simulink model "FG_costante"  (R2020a)
settings: Solver=VariableStepAuto  StartTime=0.0  StopTime=10.0  RelTol=1e-3
values from neighbouring files (symbols this model uses):
  g = 9.81    [dati_tesi_modellosimulink.m]
  L = 0.3    [dati_tesi_modellosimulink.m]
  Lc = L/2    (= 0.15)    [dati_tesi_modellosimulink.m]
  M = 4    [dati_tesi_modellosimulink.m]
  mc = 0    [dati_tesi_modellosimulink.m]
libraries: fuzblock x7, simulink x5, simulink_extras x2
settings Model: Creator=laura  LastModifiedBy=laura

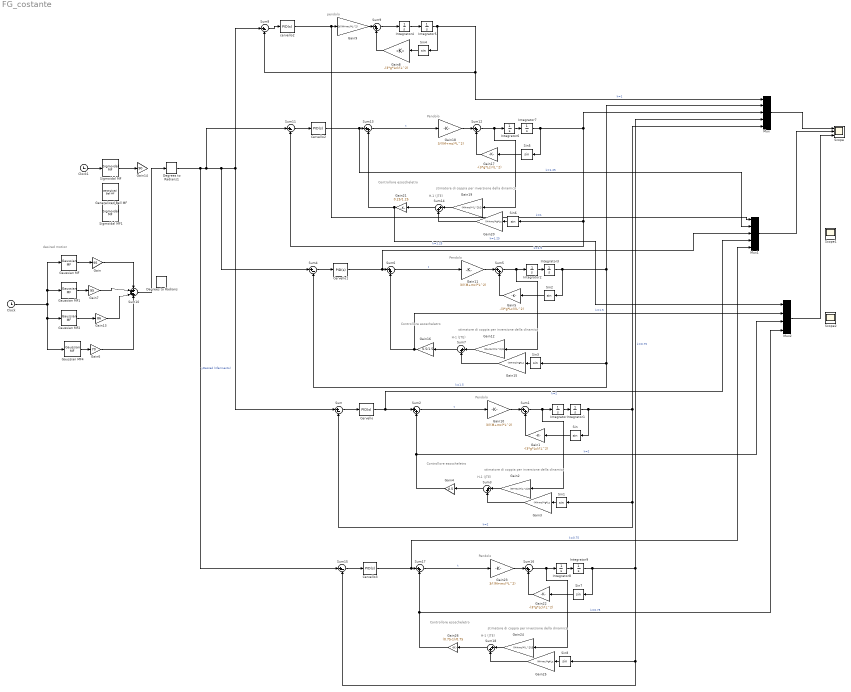
== system FG_costante ==
  note: Controllore esoscheletro
  note: stimatore di coppia per inversione della dinamica
  note: pendolo
  note: Pendolo
  note: H-1 (JTE)
  note: desired motion
  note: Pendolo
  note: H-1 (JTE)
  note: Controllore esoscheletro
  note: stimatore di coppia per inversione della dinamica
  note: Pendolo
  note: H-1 (JTE)
  note: Controllore esoscheletro
  note: stimatore di coppia per inversione della dinamica
  note: Pendolo
  note: H-1 (JTE)
  note: Controllore esoscheletro
  note: stimatore di coppia per inversione della dinamica
  Cervello{,1..3} (4 alike) : simulink/Continuous/PID Controller  Controller=PID  Form=Parallel  TimeDomain=Continuous-time  UseExternalTs=off  SampleTime=-1  IntegratorMethod=Forward Euler  FilterMethod=Forward Euler  ControllerParametersSource=internal  P=20.396  I=105.7651  D=6.3413  UseFilter=on  N=150.7964  TunerSelectOption=Transfer Function Based (PID Tuner App)  InitialConditionSource=internal  InitialConditionForIntegrator=0  InitialConditionForFilter=0  DifferentiatorICPrevScaledInput=0  ExternalReset=none  TrackingMode=off  Kt=1  LimitOutput=off  UpperSaturationLimit=inf  LowerSaturationLimit=-inf  LinearizeAsGain=on  AntiWindupMode=none  Kb=1  POutMin=[]  POutMax=[]  IOutMin=[]  IOutMax=[]  DOutMin=[]  DOutMax=[]  NOutMin=[]  NOutMax=[]  SumOutMin=[]  SumOutMax=[]  SaturationOutMin=[]  SaturationOutMax=[]  PParamMin=[]  PParamMax=[]  IParamMin=[]  IParamMax=[]  DParamMin=[]  DParamMax=[]  NParamMin=[]  NParamMax=[]  KbParamMin=[]  KbParamMax=[]  KtParamMin=[]  KtParamMax=[]  KbOutMin=[]  KbOutMax=[]  KtOutMin=[]  KtOutMax=[]  IntegratorOutMin=[]  IntegratorOutMax=[]  FilterOutMin=[]  FilterOutMax=[]  SumI1OutMin=[]  SumI1OutMax=[]  SumI2OutMin=[]  SumI2OutMax=[]  SumI3OutMin=[]  SumI3OutMax=[]  SumI4OutMin=[]  SumI4OutMax=[]  SumDOutMin=[]  SumDOutMax=[]  DifferentiatorOutMin=[]  DifferentiatorOutMax=[]  FilterDiffOutCoefMin=[]  FilterDiffOutCoefMax=[]  ReciprocalOutMin=[]  ReciprocalOutMax=[]  SumDenOutMin=[]  SumDenOutMax=[]  SumNumOutMin=[]  SumNumOutMax=[]  DivideOutMin=[]  DivideOutMax=[]  UdiffTsProdOutMin=[]  UdiffTsProdOutMax=[]  NTsProdOutMin=[]  NTsProdOutMax=[]  UintegralTsProdOutMin=[]  UintegralTsProdOutMax=[]  UngainTsProdOutMin=[]  UngainTsProdOutMax=[]  IntegratorContinuousStateAttributes=''  IntegratorStateMustResolveToSignalObject=off  IntegratorRTWStateStorageClass=Auto  FilterContinuousStateAttributes=''  FilterStateMustResolveToSignalObject=off  FilterRTWStateStorageClass=Auto  ParallelPVariant=InternalParameters  IdealPVariant=Disabled  IVariant=InternalParameters  DVariant=InternalParameters  IntegratorVariant=Continuous  SatVariant=Disabled  AWVariant=Passthrough  PCopyVariant=Disabled  TRVariant=Disabled  FdbkBlocksVariant=Forward  IdealPFdbkVariant=Disabled  SatFdbkVariant=Disabled  DerivativeFilterVariant=ContFilter  NVariant=InternalParameters  NCopyVariant=Disabled  FilterICVariant=InternalICsFilter  IntegratorICVariant=InternalICs  ExternalResetVariant=Disabled  TRSumVariant=Passthrough  SumFdbkVariant=Disabled  SumVariant=Sum_PID  TsampFilterVariant=InternalTs  TsampNgainVariant=Passthrough  TsampIntegralVariant=Passthrough
  Clock : Clock
  Clock1 : Clock
  Degrees to Radians : simulink_extras/Transformations/Degrees to Radians
  Degrees to Radians1 : simulink_extras/Transformations/Degrees to Radians
  Gain : Gain  Gain=95
  Gain{1,5,8,17,22} (5 alike) : Gain  Gain=-(3*g*Lc)/(L^2)
  Gain{9..11,18,23} (5 alike) : Gain  Gain=3/((M+mc)*L^2)
  Gain{2,12,19,24} (4 alike) : Gain  Gain=(M+mc)*(L^2)/3
  Gain13 : Gain  Gain=86
  Gain14 : Gain  Gain=90
  Gain{3,15,20,25} (4 alike) : Gain  Gain=(M+mc)*g*Lc
  Gain16 : Gain  Gain=0.5/1.5
  Gain21 : Gain  Gain=0.25/1.25
  Gain26 : Gain  Gain=(0.75-1)/0.75
  Gain4 : Gain  Gain=0.5
  Gain6 : Gain  Gain=70
  Gain7 : Gain  Gain=95
  Gaussian MF : fuzblock/Membership  Functions/Gaussian MF  sigma=0.4  mu=1.78
      settings: SourceProductBaseCode=FL
  Gaussian MF1 : fuzblock/Membership  Functions/Gaussian MF  sigma=0.4  mu=7
      settings: SourceProductBaseCode=FL
  Gaussian MF2 : fuzblock/Membership  Functions/Gaussian MF  sigma=0.38  mu=3.42
      settings: SourceProductBaseCode=FL
  Gaussian MF4 : fuzblock/Membership  Functions/Gaussian MF  sigma=0.32  mu=2.63
      settings: SourceProductBaseCode=FL
  Generalized Bell MF : fuzblock/Membership  Functions/Generalized Bell MF  a=1.5  b=4  c=6
      settings: SourceProductBaseCode=FL
  Integrator{,1..9} (10 alike) : Integrator
  Mux : Mux  Inputs=5
  Mux1 : Mux  Inputs=5
  Mux2 : Mux
  Scope : Scope  NumInputPorts=3
  Scope1 : Scope
  Scope2 : Scope
  Sigmoidal MF : fuzblock/Membership  Functions/Sigmoidal MF  a=4  c=5
      settings: SourceProductBaseCode=FL
  Sigmoidal MF1 : fuzblock/Membership  Functions/Sigmoidal MF  a=-4  c=5
      settings: SourceProductBaseCode=FL
  Sin{,1..8} (9 alike) : Trigonometry
  Sum{,4,8,11,15} (5 alike) : Sum  Inputs=|+-
  Sum{1..3,5..7,9,12..14,16..18} (13 alike) : Sum  Inputs=|++
  Sum10 : Sum  Inputs=++++
  cervello2 : simulink/Continuous/PID Controller  Controller=PID  Form=Parallel  TimeDomain=Continuous-time  UseExternalTs=off  SampleTime=-1  IntegratorMethod=Forward Euler  FilterMethod=Forward Euler  ControllerParametersSource=internal  P=20.396  I=105.7651  D=6.3413  UseFilter=on  N=150.7964  TunerSelectOption=Transfer Function Based (PID Tuner App)  InitialConditionSource=internal  InitialConditionForIntegrator=0  InitialConditionForFilter=0  DifferentiatorICPrevScaledInput=0  ExternalReset=none  TrackingMode=off  Kt=1  LimitOutput=off  UpperSaturationLimit=inf  LowerSaturationLimit=-inf  LinearizeAsGain=on  AntiWindupMode=none  Kb=1  POutMin=[]  POutMax=[]  IOutMin=[]  IOutMax=[]  DOutMin=[]  DOutMax=[]  NOutMin=[]  NOutMax=[]  SumOutMin=[]  SumOutMax=[]  SaturationOutMin=[]  SaturationOutMax=[]  PParamMin=[]  PParamMax=[]  IParamMin=[]  IParamMax=[]  DParamMin=[]  DParamMax=[]  NParamMin=[]  NParamMax=[]  KbParamMin=[]  KbParamMax=[]  KtParamMin=[]  KtParamMax=[]  KbOutMin=[]  KbOutMax=[]  KtOutMin=[]  KtOutMax=[]  IntegratorOutMin=[]  IntegratorOutMax=[]  FilterOutMin=[]  FilterOutMax=[]  SumI1OutMin=[]  SumI1OutMax=[]  SumI2OutMin=[]  SumI2OutMax=[]  SumI3OutMin=[]  SumI3OutMax=[]  SumI4OutMin=[]  SumI4OutMax=[]  SumDOutMin=[]  SumDOutMax=[]  DifferentiatorOutMin=[]  DifferentiatorOutMax=[]  FilterDiffOutCoefMin=[]  FilterDiffOutCoefMax=[]  ReciprocalOutMin=[]  ReciprocalOutMax=[]  SumDenOutMin=[]  SumDenOutMax=[]  SumNumOutMin=[]  SumNumOutMax=[]  DivideOutMin=[]  DivideOutMax=[]  UdiffTsProdOutMin=[]  UdiffTsProdOutMax=[]  NTsProdOutMin=[]  NTsProdOutMax=[]  UintegralTsProdOutMin=[]  UintegralTsProdOutMax=[]  UngainTsProdOutMin=[]  UngainTsProdOutMax=[]  IntegratorContinuousStateAttributes=''  IntegratorStateMustResolveToSignalObject=off  IntegratorRTWStateStorageClass=Auto  FilterContinuousStateAttributes=''  FilterStateMustResolveToSignalObject=off  FilterRTWStateStorageClass=Auto  ParallelPVariant=InternalParameters  IdealPVariant=Disabled  IVariant=InternalParameters  DVariant=InternalParameters  IntegratorVariant=Continuous  SatVariant=Disabled  AWVariant=Passthrough  PCopyVariant=Disabled  TRVariant=Disabled  FdbkBlocksVariant=Forward  IdealPFdbkVariant=Disabled  SatFdbkVariant=Disabled  DerivativeFilterVariant=ContFilter  NVariant=InternalParameters  NCopyVariant=Disabled  FilterICVariant=InternalICsFilter  IntegratorICVariant=InternalICs  ExternalResetVariant=Disabled  TRSumVariant=Passthrough  SumFdbkVariant=Disabled  SumVariant=Sum_PID  TsampFilterVariant=InternalTs  TsampNgainVariant=Passthrough  TsampIntegralVariant=Passthrough
  wires:
  Sum9/1 -> Integrator4/1
  Sum8/1 -> cervello2/1
  cervello2/1 -> Mux1/1, Gain9/1  "k=1"
  Sin4/1 -> Gain8/1
  Gain8/1 -> Sum9/2
  Integrator5/1 -> Mux/1, Sum8/2, Sin4/1  "k=1"
  Gain9/1 -> Sum9/1
  Integrator4/1 -> Integrator5/1
  Gain3/1 -> Sum3/2
  Sin1/1 -> Gain3/1
  Gain10/1 -> Sum1/1
  Sum2/1 -> Gain10/1  "t"
  Gain2/1 -> Sum3/1
  Integrator/1 -> Integrator1/1
  Gain1/1 -> Sum1/2
  Integrator1/1 -> Sin/1, Mux/5, Sum/2, Sin1/1  "k=2"
  Sin/1 -> Gain1/1
  Sum1/1 -> Integrator/1, Gain2/1
  Sum/1 -> Cervello/1
  Cervello/1 -> Sum2/1, Mux1/4  "k=2"
  Gain4/1 -> Sum2/2, Mux2/3  "k=2"
  Sum3/1 -> Gain4/1
  Gain7/1 -> Sum10/2
  Gain13/1 -> Sum10/3
  Gaussian MF2/1 -> Gain13/1
  Gaussian MF1/1 -> Gain7/1
  Gaussian MF/1 -> Gain/1
  Gaussian MF4/1 -> Gain6/1
  Gain6/1 -> Sum10/4
  Gain/1 -> Sum10/1
  Clock/1 -> Gaussian MF/1, Gaussian MF1/1, Gaussian MF4/1, Gaussian MF2/1
  Clock1/1 -> Sigmoidal MF/1
  Sum7/1 -> Gain16/1
  Gain16/1 -> Mux2/2, Sum6/2  "k=1.5"
  Cervello1/1 -> Mux1/3, Sum6/1  "k=1.5"
  Sum4/1 -> Cervello1/1
  Sum5/1 -> Integrator2/1, Gain12/1
  Sin2/1 -> Gain5/1
  Gain5/1 -> Sum5/2
  Integrator2/1 -> Integrator3/1
  Integrator3/1 -> Sin2/1, Mux/2, Sum4/2, Sin3/1  "k=1.5"
  Sin3/1 -> Gain15/1
  Gain15/1 -> Sum7/2
  Gain11/1 -> Sum5/1
  Sum6/1 -> Gain11/1  "t"
  Gain12/1 -> Sum7/1
  Sum14/1 -> Gain21/1
  Gain21/1 -> Mux2/1, Sum13/2  "k=1.25"
  Cervello2/1 -> Mux1/2, Sum13/1  "k=1.25"
  Sum11/1 -> Cervello2/1
  Sum12/1 -> Integrator6/1, Gain19/1
  Sin5/1 -> Gain17/1
  Gain17/1 -> Sum12/2
  Integrator6/1 -> Integrator7/1
  Integrator7/1 -> Sin5/1, Mux/3, Sum11/2, Sin6/1  "k=1.25"
  Sin6/1 -> Gain20/1
  Gain20/1 -> Sum14/2
  Gain18/1 -> Sum12/1
  Sum13/1 -> Gain18/1  "t"
  Gain19/1 -> Sum14/1
  Degrees to Radians1/1 -> Sum15/1, Sum11/1, Sum/1, Sum8/1, Sum4/1  "yDesired (riferimento)"
  Sum18/1 -> Gain26/1
  Gain26/1 -> Sum17/2, Mux2/4  "k=0.75"
  Cervello3/1 -> Mux1/5, Sum17/1  "k=0.75"
  Sum15/1 -> Cervello3/1
  Sum16/1 -> Integrator8/1, Gain24/1
  Sin7/1 -> Gain22/1
  Gain22/1 -> Sum16/2
  Integrator8/1 -> Integrator9/1
  Integrator9/1 -> Sin7/1, Mux/4, Sum15/2, Sin8/1  "k=0.75"
  Sin8/1 -> Gain25/1
  Gain25/1 -> Sum18/2
  Gain23/1 -> Sum16/1
  Sum17/1 -> Gain23/1  "t"
  Gain24/1 -> Sum18/1
  Mux1/1 -> Scope/2
  Mux2/1 -> Scope/3
  Mux/1 -> Scope/1
  Sigmoidal MF/1 -> Gain14/1
  Sum10/1 -> Degrees to Radians1/1
